simulink model "station2_task"  (Simulink 3.00)
libraries: candrvlib x1

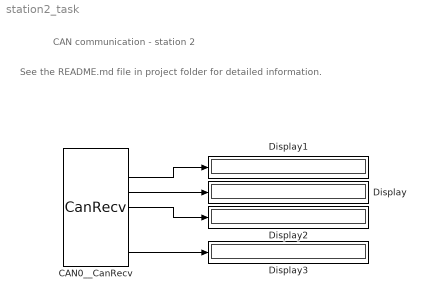
== system station2_task ==
  note: See the README.md file in project folder for detailed information.
  note: CAN communication - station 2
  CAN0__CanRecv : candrvlib/CanRecv  filterId=0x123  filterIdMask=0xFFF  filterLength=-1  RTR=off  EXT=off  timeout=10  nmax=1
  Display{,1..3} (4 alike) : Display
      Display settings: Format=hex
      Display1 settings: Format=hex
      Display2 settings: Format=hex
      Display3 settings: Format=short
  wires:
  CAN0__CanRecv/2 -> Display1/1
  CAN0__CanRecv/3 -> Display/1
  CAN0__CanRecv/4 -> Display2/1
  CAN0__CanRecv/7 -> Display3/1
